simulink model "chap13_2sim"  (Simulink 8.1)
settings: Solver=ode45  StartTime=0.0  StopTime=5  RelTol=1e-3
settings Model: Creator=ljk  LastModifiedBy=liujk  ExtModeTrigMode=oneshot  ExtModeArmWhenConnect=off
settings DataIOCC: LimitDataPoints=off  SignalLoggingName=sigsOut
settings OptimizationCC: BooleanDataType=off
settings DebuggingCC: SaveWithParameterizedLinksMsg=none  SignalResolutionControl=TryResolveAllWithWarning  SolverPrmCheckMsg=none  MultiTaskDSMMsg=warning  MultiTaskCondExecSysMsg=none
settings HardwareCC: TargetIntDivRoundTo=Zero  TargetEndianess=LittleEndian  TargetHWDeviceType=MATLAB Host  ProdEqTarget=off
settings RTWCC: IncludeERTFirstTime=on

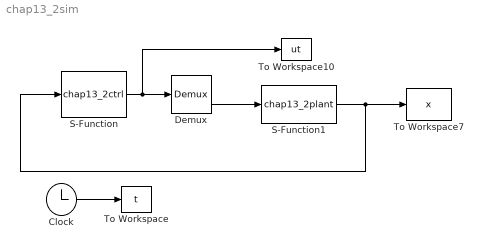
== system chap13_2sim ==
  Clock : Clock
  Demux : Demux  Outputs=3
  S-Function : S-Function  FunctionName=chap13_2ctrl  EnableBusSupport=off
  S-Function1 : S-Function  FunctionName=chap13_2plant  EnableBusSupport=off
  To Workspace : ToWorkspace  VariableName=t  SampleTime=-1
  To Workspace10 : ToWorkspace  VariableName=ut  SampleTime=-1
  To Workspace7 : ToWorkspace  VariableName=x  SampleTime=-1
  wires:
  S-Function1/1 -> S-Function/1, To Workspace7/1
  Clock/1 -> To Workspace/1
  S-Function/1 -> Demux/1, To Workspace10/1
  Demux/3 -> S-Function1/1
